simulink subsystem "Main"  (R2025b)
settings: Solver=VariableStepAuto  StartTime=0.0  StopTime=10.0  RelTol=1e-3
undefined symbols (not defined in the file): Aero_balance, Aeromaps_ON, air_density, Balance_R_11, Br_coef_of_friction_F, Br_coef_of_friction_R, Br_pistons_area_F, Br_pistons_area_R, CdA, CdA_R_11, ClA, ClA_R_11, CoG_z, Default_Fz_FL, Default_Fz_FR, Default_Fz_RL, Default_Fz_RR, Effective_br_disk_r_F, Effective_br_disk_r_R, Front_brake_balance, Front_brake_pump_area, Front_desired_brake_p_balance, Fx, Fy, Fz, g, Gear_ratio, Iz_wehicle, Iz_wheel, Lf, LLTD, Lock_brake_balance, Lr, Mass, Motor_maximum_power, PRT_efficiency, Rear_brake_pump_area, Roll_Angle_11, SA, SR, start_acc_x, start_acc_y, start_velocity_x, start_velocity_y, start_yaw_acc, start_yaw_rate, Static_Camber_FL, Static_Camber_FR, Static_Camber_RL, Static_Camber_RR, Static_Toe_FL, Static_Toe_FR, Static_Toe_RL, Static_Toe_RR, Steering_Angle_FL, Steering_Angle_FR, Steering_Wheel_Angle, Tire_pressure_FL, Tire_pressure_FR, Tire_pressure_RL ... (+18)
libraries: simulink_extras x9, simulink x7
(part 2 of 3)

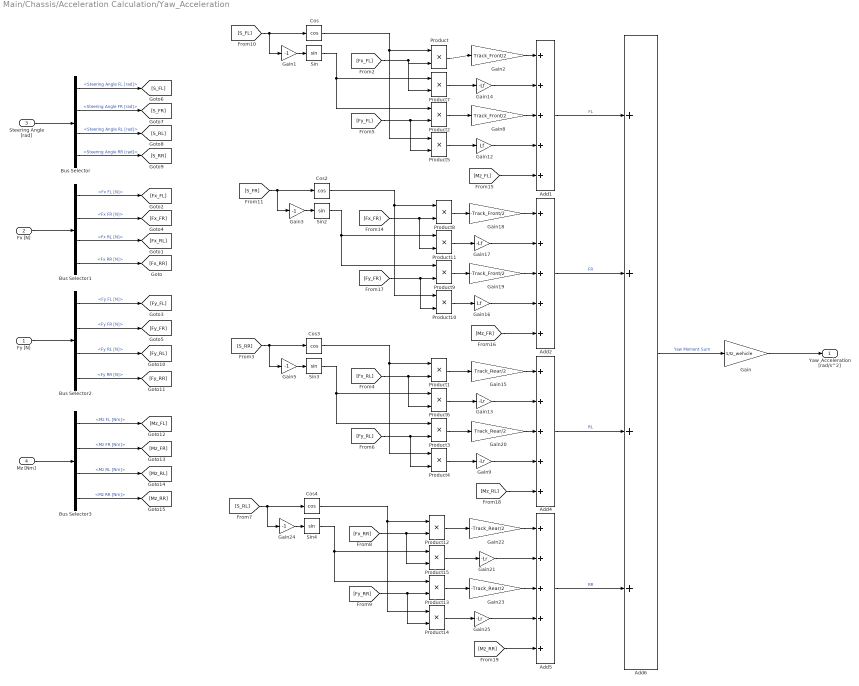
== system Main/Chassis/Acceleration Calculation/Yaw_Acceleration ==
  Fy [N] : Inport
  Fx [N] : Inport  Port=2
  Steering Angle [rad] : Inport  Port=3
  Mz [Nm] : Inport  Port=4
  Add{1..2,4..5} (4 alike) : Sum  Inputs=5
  Add6 : Sum  Inputs=4
  Bus Selector : BusSelector  OutputSignals=Steering Angle FL [rad],Steering Angle FR [rad],Steering Angle RL [rad],Steering Angle RR [rad]
  Bus Selector1 : BusSelector  OutputSignals=Fx FL [N],Fx FR [N],Fx RL [N],Fx RR [N]
  Bus Selector2 : BusSelector  OutputSignals=Fy FL [N],Fy FR [N],Fy RL [N],Fy RR [N]
  Bus Selector3 : BusSelector  OutputSignals=Mz FL [Nm],Mz FR [Nm],Mz RL [Nm],Mz RR [Nm]
  Cos{,2..4} (4 alike) : Trigonometry  Operator=cos
  Gain : Gain  Gain=1/Iz_wehicle
  Gain{1,3,5,24} (4 alike) : Gain  Gain=-1
  Gain12 : Gain  Gain=Lf
  Gain{9,13,21,25} (4 alike) : Gain  Gain=-Lr
  Gain14 : Gain  Gain=-Lf
  Gain15 : Gain  Gain=Track_Rear/2
  Gain16 : Gain  Gain=Lf
  Gain17 : Gain  Gain=-Lf
  Gain18 : Gain  Gain=-Track_Front/2
  Gain19 : Gain  Gain=-Track_Front/2
  Gain2 : Gain  Gain=Track_Front/2
  Gain20 : Gain  Gain=Track_Rear/2
  Gain22 : Gain  Gain=-Track_Rear/2
  Gain23 : Gain  Gain=-Track_Rear/2
  Gain8 : Gain  Gain=Track_Front/2
  Product{,1..15} (16 alike) : Product
  Sin{,2..4} (4 alike) : Trigonometry
  Yaw_Acceleration [rad/s^2] : Outport
  wires:
  Add1/1 -> Add6/1  "FL"
  Add5/1 -> Add6/4  "RR"
  Add2/1 -> Add6/2  "FR"
  Add4/1 -> Add6/3  "RL"
  [Mz_RR] -> Add5/5
  [Mz_RL] -> Add4/5
  [Mz_FR] -> Add2/5
  [Mz_FL] -> Add1/5
  Bus Selector3/2 -> [Mz_FR]  "<Mz FR [Nm]>"
  Bus Selector3/4 -> [Mz_RR]  "<Mz RR [Nm]>"
  Bus Selector3/3 -> [Mz_RL]  "<Mz RL [Nm]>"
  Bus Selector3/1 -> [Mz_FL]  "<Mz FL [Nm]>"
  Cos4/1 -> Product12/1, Product14/1
  Gain23/1 -> Add5/3
  [Fx_RR] -> Product12/2, Product15/2
  Gain22/1 -> Add5/1
  Gain21/1 -> Add5/2
  [Fy_RR] -> Product14/2, Product13/2
  [S_RL] -> Gain24/1, Cos4/1
  Gain25/1 -> Add5/4
  Gain24/1 -> Sin4/1
  Product13/1 -> Gain23/1
  Product12/1 -> Gain22/1
  Product14/1 -> Gain25/1
  Sin4/1 -> Product13/1, Product15/1
  Product15/1 -> Gain21/1
  Cos3/1 -> Product1/1, Product4/1
  Sin3/1 -> Product3/1, Product6/1
  Product4/1 -> Gain9/1
  Gain5/1 -> Sin3/1
  Product3/1 -> Gain20/1
  Product1/1 -> Gain15/1
  Product6/1 -> Gain13/1
  Gain9/1 -> Add4/4
  Gain20/1 -> Add4/3
  Gain13/1 -> Add4/2
  Gain15/1 -> Add4/1
  [Fx_RL] -> Product6/2, Product1/2
  [Fy_RL] -> Product4/2, Product3/2
  [S_RR] -> Cos3/1, Gain5/1
  Cos2/1 -> Product8/1, Product10/1
  Sin2/1 -> Product9/1, Product11/1
  Product10/1 -> Gain16/1
  Gain3/1 -> Sin2/1
  Product9/1 -> Gain19/1
  Product8/1 -> Gain18/1
  Product11/1 -> Gain17/1
  Gain16/1 -> Add2/4
  Gain19/1 -> Add2/3
  Gain17/1 -> Add2/2
  Gain18/1 -> Add2/1
  [Fx_FR] -> Product8/2, Product11/2
  [Fy_FR] -> Product10/2, Product9/2
  [S_FR] -> Cos2/1, Gain3/1
  Gain12/1 -> Add1/4
  Gain14/1 -> Add1/2
  Gain8/1 -> Add1/3
  Gain2/1 -> Add1/1
  Bus Selector/2 -> [S_FR]  "<Steering Angle FR [rad]>"
  [S_FL] -> Cos/1, Gain1/1
  Bus Selector/1 -> [S_FL]  "<Steering Angle FL [rad]>"
  Bus Selector/4 -> [S_RR]  "<Steering Angle RR [rad]>"
  Bus Selector/3 -> [S_RL]  "<Steering Angle RL [rad]>"
  Bus Selector2/2 -> [Fy_FR]  "<Fy FR [N]>"
  Bus Selector1/2 -> [Fx_FR]  "<Fx FR [N]>"
  [Fy_FL] -> Product5/2, Product2/2
  Bus Selector2/1 -> [Fy_FL]  "<Fy FL [N]>"
  [Fx_FL] -> Product7/2, Product/2
  Bus Selector1/1 -> [Fx_FL]  "<Fx FL [N]>"
  Mz [Nm]/1 -> Bus Selector3/1
  Product5/1 -> Gain12/1
  Sin/1 -> Product2/1, Product7/1
  Product/1 -> Gain2/1
  Product2/1 -> Gain8/1
  Bus Selector2/4 -> [Fy_RR]  "<Fy RR [N]>"
  Fx [N]/1 -> Bus Selector1/1
  Product7/1 -> Gain14/1
  Cos/1 -> Product/1, Product5/1
  Bus Selector1/3 -> [Fx_RL]  "<Fx RL [N]>"
  Fy [N]/1 -> Bus Selector2/1
  Bus Selector2/3 -> [Fy_RL]  "<Fy RL [N]>"
  Gain1/1 -> Sin/1
  Steering Angle [rad]/1 -> Bus Selector/1
  Bus Selector1/4 -> [Fx_RR]  "<Fx RR [N]>"
  Add6/1 -> Gain/1  "Yaw Moment Sum"
  Gain/1 -> Yaw_Acceleration [rad/s^2]/1

== system Main/Powertrain/Motors/Control Algorithms ==
  Motor Torque after FW [Nm] : Inport
  Torque Command [Nm] : Inport  Port=2
  Wheel Speed [rad/s] : Inport  Port=3
  Bus Creator : BusCreator  Inputs=4
  Bus Selector : BusSelector  OutputSignals=Motor Torque FL after FW [Nm],Motor Torque FR after FW [Nm],Motor Torque RL after FW [Nm],Motor Torque RR after FW [Nm]
  Constant : Constant  Value=TV_ON
  Gain : Gain
  Gain1 : Gain
  Switch{,1..3} (4 alike) : Switch  Criteria=u2 > Threshold  SaturateOnIntegerOverflow=off  InputSameDT=off
  TV Algorithm : Subsystem
  Motor Torque after TV [Nm] : Outport
  wires:
  Wheel Speed [rad/s]/1 -> TV Algorithm/2(Wheel Speed [rad/s])
  Gain1/1 -> Switch3/3
  Gain/1 -> Switch2/3
  Torque Command [Nm]/1 -> TV Algorithm/1(Torque Command [Nm])
  TV Algorithm/4(Commanded Torque RR [Nm]) -> Switch3/1  "Motor Torque RR"
  TV Algorithm/3(Commanded Torque RL [Nm]) -> Switch2/1  "Motor Torque RL"
  TV Algorithm/2(Commanded Torque FR [Nm]) -> Switch1/1
  TV Algorithm/1(Commanded Torque FL [Nm]) -> Switch/1
  Switch1/1 -> Bus Creator/2  "Motor Torque FR after TV [Nm]"
  Switch/1 -> Bus Creator/1  "Motor Torque FL after TV [Nm]"
  Bus Creator/1 -> Motor Torque after TV [Nm]/1  "Motor Torque after TV [Nm]"
  Switch2/1 -> Bus Creator/3  "Motor Torque RL after TV [Nm]"
  Switch3/1 -> Bus Creator/4  "Motor Torque RR after TV [Nm]"
  Bus Selector/4 -> Gain1/1  "<Motor Torque RR after FW [Nm]>"
  Bus Selector/3 -> Gain/1  "<Motor Torque RL after FW [Nm]>"
  Bus Selector/2 -> Switch1/3  "<Motor Torque FR after FW [Nm]>"
  Bus Selector/1 -> Switch/3  "<Motor Torque FL after FW [Nm]>"
  Motor Torque after FW [Nm]/1 -> Bus Selector/1
  Constant/1 -> Switch/2, Switch1/2, Switch2/2, Switch3/2

== system Main/Powertrain/Motors/Field Weakening ==
  Torque Command [Nm] : Inport
  Wheel Speed [rad/s] : Inport  Port=2
  Bus Creator : BusCreator  Inputs=4
  Bus Selector : BusSelector  OutputSignals=Wheel Speed FL [rad/s],Wheel Speed FR [rad/s],Wheel Speed RL [rad/s],Wheel Speed RR [rad/s]
  Constant : Constant  Value=Motor_maximum_power
  Gain : Gain  Gain=0
  Gain{1..2,5,7} (4 alike) : Gain  Gain=-1
  Gain10 : Gain
  Gain11 : Gain
  Gain{3..4,6,8} (4 alike) : Gain  Gain=Gear_ratio
  Gain9 : Gain  Gain=0
  Product : Product  Inputs=*/
  Product1 : Product  Inputs=/*
  Product2 : Product  Inputs=/*
  Product3 : Product  Inputs=*/
  Saturation Dynamic{,1..3} (4 alike) : simulink/Discontinuities/Saturation Dynamic  OutMin=[]  OutMax=[]  OutDataTypeStr=Inherit: Same as second input  OutDataType=fixdt(1, 16)  OutScaling=2^-10  DoSatur=off
  Motor Torque after FW [Nm] : Outport
  wires:
  Gain2/1 -> Saturation Dynamic1/3
  Gain1/1 -> Saturation Dynamic/3
  Wheel Speed [rad/s]/1 -> Bus Selector/1
  Gain11/1 -> Bus Creator/2  "Motor Torque RL after FW [Nm]"
  Gain10/1 -> Bus Creator/3  "Motor Torque RR after FW [Nm]"
  Gain9/1 -> Bus Creator/4  "Motor Torque FR after FW [Nm]"
  Gain/1 -> Bus Creator/1  "Motor Torque FL after FW [Nm]"
  Bus Creator/1 -> Motor Torque after FW [Nm]/1  "Motor Torque after FW [Nm]"
  Saturation Dynamic3/1 -> Gain9/1
  Gain7/1 -> Saturation Dynamic3/3
  Product3/1 -> Saturation Dynamic3/1, Gain7/1  "Maximum Torque FR after FW [Nm]"
  Bus Selector/4 -> Gain8/1  "<Wheel Speed RR [rad/s]>"
  Gain8/1 -> Product3/2  "Motor Speed FR [rad/s]"
  Constant/1 -> Product3/1, Product/1, Product2/2, Product1/2
  Torque Command [Nm]/1 -> Saturation Dynamic1/2, Saturation Dynamic3/2, Saturation Dynamic/2, Saturation Dynamic2/2
  Gain5/1 -> Saturation Dynamic2/3
  Bus Selector/1 -> Gain6/1  "<Wheel Speed FL [rad/s]>"
  Product2/1 -> Saturation Dynamic2/1, Gain5/1  "Maximum Torque FL after FW [Nm]"
  Gain6/1 -> Product2/1  "Motor Speed FL [rad/s]"
  Saturation Dynamic2/1 -> Gain/1
  Saturation Dynamic/1 -> Gain11/1
  Gain4/1 -> Product/2  "Motor Speed RR [rad/s]"
  Gain3/1 -> Product1/1  "Motor Speed RL [rad/s]"
  Bus Selector/3 -> Gain4/1  "<Wheel Speed RL [rad/s]>"
  Product1/1 -> Gain1/1, Saturation Dynamic/1  "Maximum Torque RL after FW [Nm]"
  Bus Selector/2 -> Gain3/1  "<Wheel Speed FR [rad/s]>"
  Product/1 -> Gain2/1, Saturation Dynamic1/1  "Maximum Torque RR after FW [Nm]"
  Saturation Dynamic1/1 -> Gain10/1

== system Main/Powertrain/Motors/Power Limit ==
  Motor Torque after TV [Nm] : Inport
  "Torque Command {Nm]" : Inport  Port=2
  Wheel Speed [rad/s] : Inport  Port=3
  Bus Creator : BusCreator  Inputs=5
  Bus Selector : BusSelector  OutputSignals=Motor Torque FL after TV [Nm],Motor Torque FR after TV [Nm],Motor Torque RL after TV [Nm],Motor Torque RR after TV [Nm]
  Constant : Constant  Value=TV_ON
  Power Calculation : Subsystem
  Switch{,1..3} (4 alike) : Switch  Criteria=u2 > Threshold  SaturateOnIntegerOverflow=off  InputSameDT=off
  Motor Power [W] : Outport
  Motor Torque [Nm] : Outport  Port=2
  wires:
  Wheel Speed [rad/s]/1 -> Power Calculation/1(Wheel Speed [rad/s])
  "Torque Command {Nm]"/1 -> Bus Creator/5
  Bus Creator/1 -> Motor Torque [Nm]/1
  Constant/1 -> Switch1/2, Switch3/2, Switch2/2, Switch/2
  Bus Selector/1 -> Switch/3, Switch/1  "<Motor Torque FL after TV [Nm]>"
  Bus Selector/4 -> Switch3/3, Switch3/1  "<Motor Torque RR after TV [Nm]>"
  Bus Selector/3 -> Switch2/3, Switch2/1  "<Motor Torque RL after TV [Nm]>"
  Switch1/1 -> Bus Creator/2  "Motor Torque FR [Nm]"
  Switch/1 -> Bus Creator/1  "Motor Torque FL [Nm]"
  Switch2/1 -> Bus Creator/3  "Motor Torque RL [Nm]"
  Switch3/1 -> Bus Creator/4  "Motor Torque RR [Nm]"
  Bus Selector/2 -> Switch1/3, Switch1/1  "<Motor Torque FR after TV [Nm]>"
  Power Calculation/1(Motor Power [W]) -> Motor Power [W]/1
  Motor Torque after TV [Nm]/1 -> Power Calculation/2(Motor Torque after TV [Nm]), Bus Selector/1

== system Main/Powertrain/Motors/Regen Braking ==
  Brake Pressure Front [bar] : Inport
  Brake Pressure Rear [bar] : Inport  Port=2
  " " : Constant  Value=Front_desired_brake_p_balance
  AND : Logic  IconShape=distinctive  AllPortsSameDT=off  OutDataTypeStr=boolean
  Cast To Boolean : DataTypeConversion  OutDataTypeStr=double  SaturateOnIntegerOverflow=off  RndMeth=Floor
  Compare To Constant : simulink/Logic and Bit Operations/Compare To Constant  relop=>=  const=5  OutDataTypeStr=boolean
  Compare To Constant1 : simulink/Logic and Bit Operations/Compare To Constant  relop=>=  const=5  OutDataTypeStr=boolean
  Gain : Gain  Gain=-1
  Product1 : Product
  Saturation2 : Saturate  UpperLimit=29  LowerLimit=0
  Subsystem : Subsystem
  Torque_to_Current_Conversion : Lookup_n-D  NumberOfTableDimensions=1  BreakpointsForDimension1=[0 29]  Table=[0 44]  InternalRulePriority=Speed  RndMeth=Simplest
  Negative Torque Command [Nm] : Outport
  wires:
  Brake Pressure Front [bar]/1 -> Subsystem/1(Brake_Preasure_Front), Compare To Constant1/1
  Brake Pressure Rear [bar]/1 -> Subsystem/2(Brake_Preasure_Rear), Compare To Constant/1
  Gain/1 -> Negative Torque Command [Nm]/1  "Negative Torque Command [Nm]"
  Compare To Constant1/1 -> AND/1
  AND/1 -> Cast To Boolean/1
  Subsystem/1("Motor_Rear_\"Preasure\"") -> Torque_to_Current_Conversion/1
  Saturation2/1 -> Product1/2
  Product1/1 -> Gain/1
  Torque_to_Current_Conversion/1 -> Saturation2/1
  Cast To Boolean/1 -> Product1/1
  Compare To Constant/1 -> AND/2
  " "/1 -> Subsystem/3(Desired_Brake_Balance)  "Desired_Brake_Balance"

== system Main/Powertrain/Motors/Torque Command [Nm] ==
  APPS [%] : Inport
  Constant : Constant  Value=Torque_limit_set
  Merge : Merge  Inputs=11
  Switch Case : SwitchCase  CaseConditions={1,2,3,4,5,6,7,8,9,10}
  Switch Case Action Subsystem : Subsystem  TreatAsAtomicUnit=on
  Switch Case Action Subsystem1 : Subsystem  TreatAsAtomicUnit=on
  Switch Case Action Subsystem10 : Subsystem  TreatAsAtomicUnit=on
  Switch Case Action Subsystem2 : Subsystem  TreatAsAtomicUnit=on
  Switch Case Action Subsystem3 : Subsystem  TreatAsAtomicUnit=on
  Switch Case Action Subsystem4 : Subsystem  TreatAsAtomicUnit=on
  Switch Case Action Subsystem5 : Subsystem  TreatAsAtomicUnit=on
  Switch Case Action Subsystem6 : Subsystem  TreatAsAtomicUnit=on
  Switch Case Action Subsystem7 : Subsystem  TreatAsAtomicUnit=on
  Switch Case Action Subsystem8 : Subsystem  TreatAsAtomicUnit=on
  Switch Case Action Subsystem9 : Subsystem  TreatAsAtomicUnit=on
  Positive Torque Command [Nm] : Outport
  wires:
  Switch Case/8 -> Switch Case Action Subsystem3/Action
  Switch Case/3 -> Switch Case Action Subsystem8/Action
  Switch Case/4 -> Switch Case Action Subsystem7/Action
  Switch Case/5 -> Switch Case Action Subsystem6/Action
  Switch Case/10 -> Switch Case Action Subsystem1/Action
  Switch Case Action Subsystem/1(Out1) -> Merge/11
  Switch Case Action Subsystem2/1(Out1) -> Merge/9
  Switch Case Action Subsystem5/1(Out1) -> Merge/6
  Switch Case/6 -> Switch Case Action Subsystem5/Action
  Switch Case Action Subsystem3/1(Out1) -> Merge/8
  Switch Case Action Subsystem4/1(Out1) -> Merge/7
  Switch Case Action Subsystem6/1(Out1) -> Merge/5
  Switch Case Action Subsystem10/1(Out1) -> Merge/1
  Switch Case Action Subsystem9/1(Out1) -> Merge/2
  Switch Case/11 -> Switch Case Action Subsystem/Action
  Constant/1 -> Switch Case/1
  Switch Case/7 -> Switch Case Action Subsystem4/Action
  Switch Case Action Subsystem7/1(Out1) -> Merge/4
  Switch Case/9 -> Switch Case Action Subsystem2/Action
  Switch Case Action Subsystem1/1(Out1) -> Merge/10
  Merge/1 -> Positive Torque Command [Nm]/1
  Switch Case/1 -> Switch Case Action Subsystem10/Action
  Switch Case Action Subsystem8/1(Out1) -> Merge/3
  Switch Case/2 -> Switch Case Action Subsystem9/Action
  APPS [%]/1 -> Switch Case Action Subsystem/1(APPS), Switch Case Action Subsystem1/1(APPS), Switch Case Action Subsystem3/1(APPS), Switch Case Action Subsystem5/1(APPS), Switch Case Action Subsystem6/1(APPS), Switch Case Action Subsystem8/1(APPS), Switch Case Action Subsystem10/1(APPS), Switch Case Action Subsystem9/1(APPS), Switch Case Action Subsystem7/1(APPS), Switch Case Action Subsystem4/1(APPS), Switch Case Action Subsystem2/1(APPS)

== system Main/Wheels & Tires/Brakes/Brake_Balance_Adjustment ==
  Braking_Torque_F [Nm] : Inport
  Braking_Torque_R [Nm] : Inport  Port=2
  Add : Sum
  Add1 : Sum
  Add2 : Sum
  Compare To Constant1 : simulink/Logic and Bit Operations/Compare To Constant  relop=>  const=1  OutDataTypeStr=boolean
  Constant : Constant  Value=Lock_brake_balance
  Constant1 : Constant  Value=Lock_brake_balance
  Constant2 : Constant  Value=Front_brake_balance
  Enabled Subsystem : Subsystem  TreatAsAtomicUnit=on
  Product : Product  Inputs=*/
  Product1 : Product
  Subtract : Sum  Inputs=-+
  Subtract1 : Sum  Inputs=-+
  Switch : Switch  Threshold=1  SaturateOnIntegerOverflow=off  InputSameDT=off
  Switch1 : Switch  Threshold=1  SaturateOnIntegerOverflow=off  InputSameDT=off
  Terminator : Terminator
  Adj_Braking_Torque_F [Nm] : Outport
  Adj_Braking_Torque_R [Nm] : Outport  Port=2
  wires:
  Subtract/1 -> Switch1/3  "Locked_Torque_R"
  Add1/1 -> Switch/3  "Locked_Torque_F"
  Subtract1/1 -> Switch1/1  "Adjusted_Torque_R"
  Add2/1 -> Subtract1/2, Product1/2
  Braking_Torque_R [Nm]/1 -> Subtract/2, Add2/2
  Product1/1 -> Switch/1, Add1/2, Subtract/1, Subtract1/1  "Adjusted_Torque_F"
  Braking_Torque_F [Nm]/1 -> Add2/1, Add1/1
  Constant2/1 -> Product1/1
  Compare To Constant1/1 -> Enabled Subsystem/Enable
  Enabled Subsystem/1(Out1) -> Terminator/1  "Brake_balance"
  Product/1 -> Enabled Subsystem/1(In1)  "Brake_balance"
  Add/1 -> Product/2
  Constant1/1 -> Switch1/2
  Switch1/1 -> Adj_Braking_Torque_R [Nm]/1, Compare To Constant1/1, Add/2  "Adj_Rear"
  Switch/1 -> Add/1, Product/1, Adj_Braking_Torque_F [Nm]/1  "Adj_Front"
  Constant/1 -> Switch/2

== system Main/Wheels & Tires/Brakes/Braking_Torque_Front ==
  Brake_Pressure [bar] : Inport
  Gain : Gain  Gain=1e5
  Gain1 : Gain  Gain=Effective_br_disk_r_F
  Product : Product  Inputs=3
  coefficient of friction : Constant  Value=Br_coef_of_friction_F
  piston area : Constant  Value=Br_pistons_area_F
  Braking_torque [Nm] : Outport
  wires:
  Gain1/1 -> Braking_torque [Nm]/1  "Braking torque [Nm]"
  Product/1 -> Gain1/1  "Braking force [N]"
  piston area/1 -> Product/3
  coefficient of friction/1 -> Product/2
  Gain/1 -> Product/1  "[Pa]"
  Brake_Pressure [bar]/1 -> Gain/1  "[bar]"

== system Main/Wheels & Tires/Brakes/Braking_Torque_Rear ==
  Brake_Pressure [bar] : Inport
  Gain1 : Gain  Gain=1e5
  Gain2 : Gain  Gain=Effective_br_disk_r_R
  Product2 : Product  Inputs=3
  coefficient of friction : Constant  Value=Br_coef_of_friction_R
  piston area : Constant  Value=Br_pistons_area_R
  Braking_Torque [Nm] : Outport
  wires:
  Brake_Pressure [bar]/1 -> Gain1/1
  coefficient of friction/1 -> Product2/2
  Gain1/1 -> Product2/1  "[Pa]"
  Gain2/1 -> Braking_Torque [Nm]/1  "Braking_Torque [Nm]"
  piston area/1 -> Product2/3
  Product2/1 -> Gain2/1  "Braking_Force [N]"

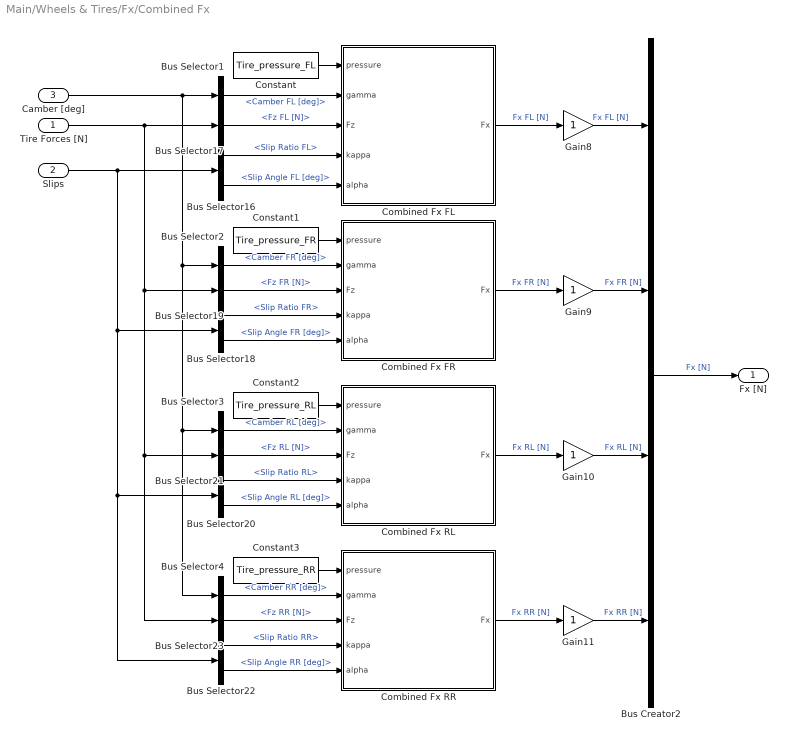
== system Main/Wheels & Tires/Fx/Combined Fx ==
  Tire Forces [N] : Inport
  Slips : Inport  Port=2
  Camber [deg] : Inport  Port=3
  Bus Creator2 : BusCreator  Inputs=4
  Bus Selector1 : BusSelector  OutputSignals=Camber FL [deg]
  Bus Selector16 : BusSelector  OutputSignals=Slip Ratio.Slip Ratio FL,Slip Angle [deg].Slip Angle FL [deg]
  Bus Selector17 : BusSelector  OutputSignals=Fz FL [N]
  Bus Selector18 : BusSelector  OutputSignals=Slip Ratio.Slip Ratio FR,Slip Angle [deg].Slip Angle FR [deg]
  Bus Selector19 : BusSelector  OutputSignals=Fz FR [N]
  Bus Selector2 : BusSelector  OutputSignals=Camber FR [deg]
  Bus Selector20 : BusSelector  OutputSignals=Slip Ratio.Slip Ratio RL,Slip Angle [deg].Slip Angle RL [deg]
  Bus Selector21 : BusSelector  OutputSignals=Fz RL [N]
  Bus Selector22 : BusSelector  OutputSignals=Slip Ratio.Slip Ratio RR,Slip Angle [deg].Slip Angle RR [deg]
  Bus Selector23 : BusSelector  OutputSignals=Fz RR [N]
  Bus Selector3 : BusSelector  OutputSignals=Camber RL [deg]
  Bus Selector4 : BusSelector  OutputSignals=Camber RR [deg]
  Combined Fx FL : MATLAB Function  TreatAsAtomicUnit=on
  Combined Fx FR : MATLAB Function  TreatAsAtomicUnit=on
  Combined Fx RL : MATLAB Function  TreatAsAtomicUnit=on
  Combined Fx RR : MATLAB Function  TreatAsAtomicUnit=on
  Constant : Constant  Value=Tire_pressure_FL
  Constant1 : Constant  Value=Tire_pressure_FR
  Constant2 : Constant  Value=Tire_pressure_RL
  Constant3 : Constant  Value=Tire_pressure_RR
  Gain{8..11} (4 alike) : Gain
  Fx [N] : Outport
  wires:
  Bus Selector4/1 -> Combined Fx RR/2(gamma)  "<Camber RR [deg]>"
  Bus Selector3/1 -> Combined Fx RL/2(gamma)  "<Camber RL [deg]>"
  Bus Selector2/1 -> Combined Fx FR/2(gamma)  "<Camber FR [deg]>"
  Bus Selector1/1 -> Combined Fx FL/2(gamma)  "<Camber FL [deg]>"
  Constant3/1 -> Combined Fx RR/1(pressure)
  Constant2/1 -> Combined Fx RL/1(pressure)
  Constant1/1 -> Combined Fx FR/1(pressure)
  Constant/1 -> Combined Fx FL/1(pressure)
  Camber [deg]/1 -> Bus Selector1/1, Bus Selector2/1, Bus Selector3/1, Bus Selector4/1
  Bus Creator2/1 -> Fx [N]/1  "Fx [N]"
  Bus Selector22/2 -> Combined Fx RR/5(alpha)  "<Slip Angle RR [deg]>"
  Bus Selector23/1 -> Combined Fx RR/3(Fz)  "<Fz RR [N]>"
  Bus Selector16/2 -> Combined Fx FL/5(alpha)  "<Slip Angle FL [deg]>"
  Bus Selector18/2 -> Combined Fx FR/5(alpha)  "<Slip Angle FR [deg]>"
  Bus Selector21/1 -> Combined Fx RL/3(Fz)  "<Fz RL [N]>"
  Combined Fx RL/1(Fx) -> Gain10/1  "Fx RL [N]"
  Combined Fx FL/1(Fx) -> Gain8/1  "Fx FL [N]"
  Combined Fx FR/1(Fx) -> Gain9/1  "Fx FR [N]"
  Combined Fx RR/1(Fx) -> Gain11/1  "Fx RR [N]"
  Bus Selector19/1 -> Combined Fx FR/3(Fz)  "<Fz FR [N]>"
  Gain10/1 -> Bus Creator2/3  "Fx RL [N]"
  Bus Selector16/1 -> Combined Fx FL/4(kappa)  "<Slip Ratio FL>"
  Gain8/1 -> Bus Creator2/1  "Fx FL [N]"
  Tire Forces [N]/1 -> Bus Selector23/1, Bus Selector21/1, Bus Selector19/1, Bus Selector17/1
  Bus Selector17/1 -> Combined Fx FL/3(Fz)  "<Fz FL [N]>"
  Bus Selector22/1 -> Combined Fx RR/4(kappa)  "<Slip Ratio RR>"
  Bus Selector18/1 -> Combined Fx FR/4(kappa)  "<Slip Ratio FR>"
  Bus Selector20/1 -> Combined Fx RL/4(kappa)  "<Slip Ratio RL>"
  Bus Selector20/2 -> Combined Fx RL/5(alpha)  "<Slip Angle RL [deg]>"
  Slips/1 -> Bus Selector22/1, Bus Selector20/1, Bus Selector18/1, Bus Selector16/1
  Gain9/1 -> Bus Creator2/2  "Fx FR [N]"
  Gain11/1 -> Bus Creator2/4  "Fx RR [N]"

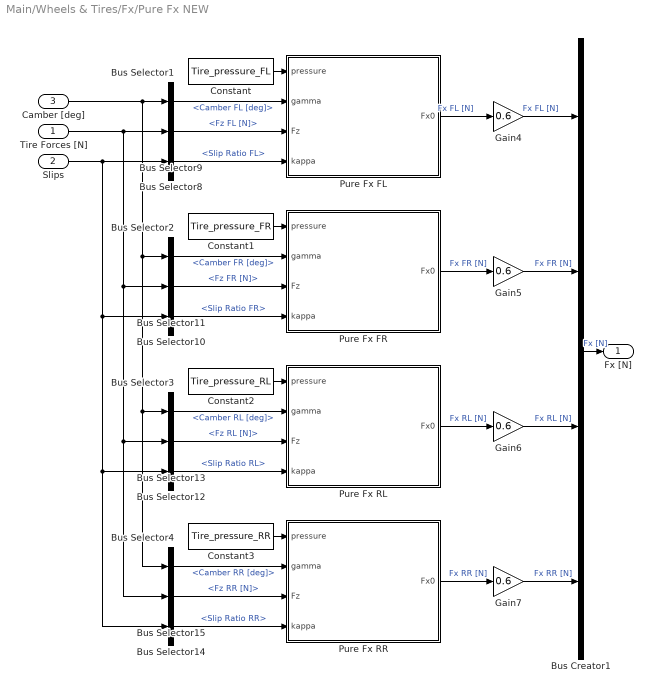
== system Main/Wheels & Tires/Fx/Pure Fx NEW ==
  Tire Forces [N] : Inport
  Slips : Inport  Port=2
  Camber [deg] : Inport  Port=3
  Bus Creator1 : BusCreator  Inputs=4
  Bus Selector1 : BusSelector  OutputSignals=Camber FL [deg]
  Bus Selector10 : BusSelector  OutputSignals=Slip Ratio.Slip Ratio FR
  Bus Selector11 : BusSelector  OutputSignals=Fz FR [N]
  Bus Selector12 : BusSelector  OutputSignals=Slip Ratio.Slip Ratio RL
  Bus Selector13 : BusSelector  OutputSignals=Fz RL [N]
  Bus Selector14 : BusSelector  OutputSignals=Slip Ratio.Slip Ratio RR
  Bus Selector15 : BusSelector  OutputSignals=Fz RR [N]
  Bus Selector2 : BusSelector  OutputSignals=Camber FR [deg]
  Bus Selector3 : BusSelector  OutputSignals=Camber RL [deg]
  Bus Selector4 : BusSelector  OutputSignals=Camber RR [deg]
  Bus Selector8 : BusSelector  OutputSignals=Slip Ratio.Slip Ratio FL
  Bus Selector9 : BusSelector  OutputSignals=Fz FL [N]
  Constant : Constant  Value=Tire_pressure_FL
  Constant1 : Constant  Value=Tire_pressure_FR
  Constant2 : Constant  Value=Tire_pressure_RL
  Constant3 : Constant  Value=Tire_pressure_RR
  Gain{4..7} (4 alike) : Gain  Gain=0.6
  Pure Fx FL : MATLAB Function  TreatAsAtomicUnit=on
  Pure Fx FR : MATLAB Function  TreatAsAtomicUnit=on
  Pure Fx RL : MATLAB Function  TreatAsAtomicUnit=on
  Pure Fx RR : MATLAB Function  TreatAsAtomicUnit=on
  Fx [N] : Outport
  wires:
  Bus Selector4/1 -> Pure Fx RR/2(gamma)  "<Camber RR [deg]>"
  Bus Selector3/1 -> Pure Fx RL/2(gamma)  "<Camber RL [deg]>"
  Bus Selector2/1 -> Pure Fx FR/2(gamma)  "<Camber FR [deg]>"
  Camber [deg]/1 -> Bus Selector1/1, Bus Selector2/1, Bus Selector3/1, Bus Selector4/1
  Bus Selector1/1 -> Pure Fx FL/2(gamma)  "<Camber FL [deg]>"
  Constant3/1 -> Pure Fx RR/1(pressure)
  Constant2/1 -> Pure Fx RL/1(pressure)
  Constant1/1 -> Pure Fx FR/1(pressure)
  Constant/1 -> Pure Fx FL/1(pressure)
  Gain6/1 -> Bus Creator1/3  "Fx RL [N]"
  Pure Fx RL/1(Fx0) -> Gain6/1  "Fx RL [N]"
  Gain7/1 -> Bus Creator1/4  "Fx RR [N]"
  Pure Fx FL/1(Fx0) -> Gain4/1  "Fx FL [N]"
  Bus Selector9/1 -> Pure Fx FL/3(Fz)  "<Fz FL [N]>"
  Bus Selector12/1 -> Pure Fx RL/4(kappa)  "<Slip Ratio RL>"
  Bus Creator1/1 -> Fx [N]/1  "Fx [N]"
  Bus Selector13/1 -> Pure Fx RL/3(Fz)  "<Fz RL [N]>"
  Gain5/1 -> Bus Creator1/2  "Fx FR [N]"
  Bus Selector10/1 -> Pure Fx FR/4(kappa)  "<Slip Ratio FR>"
  Gain4/1 -> Bus Creator1/1  "Fx FL [N]"
  Bus Selector11/1 -> Pure Fx FR/3(Fz)  "<Fz FR [N]>"
  Bus Selector14/1 -> Pure Fx RR/4(kappa)  "<Slip Ratio RR>"
  Bus Selector15/1 -> Pure Fx RR/3(Fz)  "<Fz RR [N]>"
  Tire Forces [N]/1 -> Bus Selector9/1, Bus Selector11/1, Bus Selector13/1, Bus Selector15/1
  Pure Fx RR/1(Fx0) -> Gain7/1  "Fx RR [N]"
  Pure Fx FR/1(Fx0) -> Gain5/1  "Fx FR [N]"
  Slips/1 -> Bus Selector8/1, Bus Selector12/1, Bus Selector14/1, Bus Selector10/1
  Bus Selector8/1 -> Pure Fx FL/4(kappa)  "<Slip Ratio FL>"

== system Main/Wheels & Tires/Fx/Pure Fx OLD ==
  Tire Forces [N] : Inport
  Slips : Inport  Port=2
  2-D Lookup Table1 : Lookup_n-D  BreakpointsForDimension1=Fz  BreakpointsForDimension2=SR  Table=Fx  UseLastTableValue=on  ApplyAccurateEfficientRounding=on  InternalRulePriority=Speed  RndMeth=Simplest
      settings: InputPortMap=u0,u1
  2-D Lookup Table2 : Lookup_n-D  BreakpointsForDimension1=Fz  BreakpointsForDimension2=SR  Table=Fx  UseLastTableValue=on  ApplyAccurateEfficientRounding=on  InternalRulePriority=Speed  RndMeth=Simplest
      settings: InputPortMap=u0,u1
  2-D Lookup Table3 : Lookup_n-D  BreakpointsForDimension1=Fz  BreakpointsForDimension2=SR  Table=Fx  ExtrapMethod=Clip  UseLastTableValue=on  ApplyAccurateEfficientRounding=on  InternalRulePriority=Speed  RndMeth=Simplest
      settings: InputPortMap=u0,u1
  2-D Lookup Table4 : Lookup_n-D  BreakpointsForDimension1=Fz  BreakpointsForDimension2=SR  Table=Fx  ExtrapMethod=Clip  UseLastTableValue=on  ApplyAccurateEfficientRounding=on  InternalRulePriority=Speed  RndMeth=Simplest
      settings: InputPortMap=u0,u1
  Bus Creator : BusCreator  Inputs=4
  Bus Selector : BusSelector  OutputSignals=Slip Ratio.Slip Ratio FL
  Bus Selector1 : BusSelector  OutputSignals=Fz FL [N]
  Bus Selector2 : BusSelector  OutputSignals=Slip Ratio.Slip Ratio FR
  Bus Selector3 : BusSelector  OutputSignals=Fz FR [N]
  Bus Selector4 : BusSelector  OutputSignals=Slip Ratio.Slip Ratio RL
  Bus Selector5 : BusSelector  OutputSignals=Fz RL [N]
  Bus Selector6 : BusSelector  OutputSignals=Slip Ratio.Slip Ratio RR
  Bus Selector7 : BusSelector  OutputSignals=Fz RR [N]
  Gain : Gain  Gain=0.8
  Gain1 : Gain  Gain=0.8
  Gain2 : Gain  Gain=1.6
  Gain3 : Gain  Gain=1.6
  Fx [N] : Outport
  wires:
  Bus Creator/1 -> Fx [N]/1  "Fx [N]"
  Gain2/1 -> Bus Creator/3  "Fx RL [N]"
  Bus Selector7/1 -> 2-D Lookup Table4/1  "<Fz RR [N]>"
  Bus Selector6/1 -> 2-D Lookup Table4/2  "<Slip Ratio RR>"
  Bus Selector4/1 -> 2-D Lookup Table3/2  "<Slip Ratio RL>"
  Bus Selector3/1 -> 2-D Lookup Table2/1  "<Fz FR [N]>"
  Slips/1 -> Bus Selector/1, Bus Selector2/1, Bus Selector4/1, Bus Selector6/1
  2-D Lookup Table1/1 -> Gain/1  "Fx FL [N]"
  Bus Selector1/1 -> 2-D Lookup Table1/1  "<Fz FL [N]>"
  Bus Selector/1 -> 2-D Lookup Table1/2  "<Slip Ratio FL>"
  2-D Lookup Table4/1 -> Gain3/1  "Fx RR [N]"
  Bus Selector5/1 -> 2-D Lookup Table3/1  "<Fz RL [N]>"
  Gain/1 -> Bus Creator/1  "Fx FL [N]"
  Gain1/1 -> Bus Creator/2  "Fx FR [N]"
  Bus Selector2/1 -> 2-D Lookup Table2/2  "<Slip Ratio FR>"
  Tire Forces [N]/1 -> Bus Selector3/1, Bus Selector5/1, Bus Selector7/1, Bus Selector1/1
  Gain3/1 -> Bus Creator/4  "Fx RR [N]"
  2-D Lookup Table3/1 -> Gain2/1  "Fx RL [N]"
  2-D Lookup Table2/1 -> Gain1/1  "Fx FR [N]"

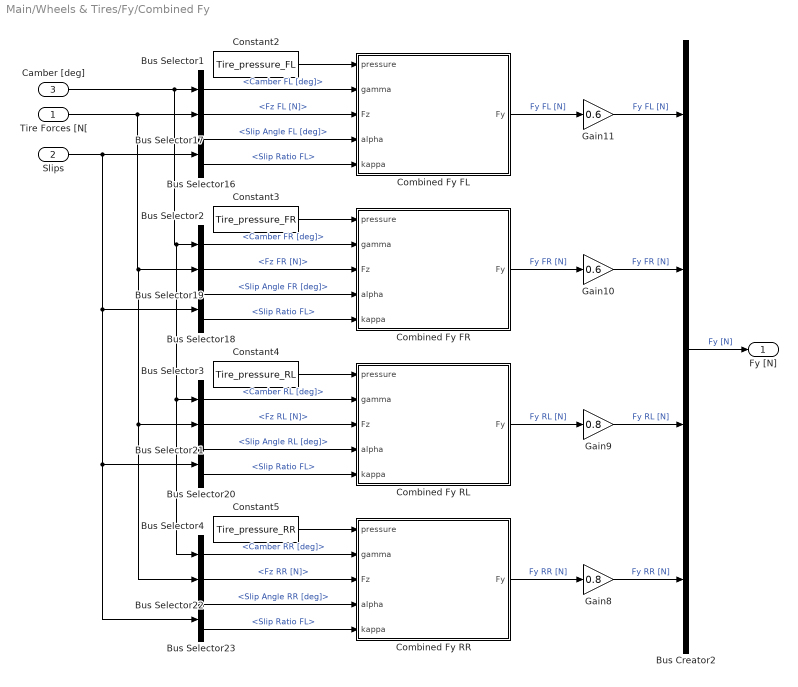
== system Main/Wheels & Tires/Fy/Combined Fy ==
  Tire Forces [N[ : Inport
  Slips : Inport  Port=2
  Camber [deg] : Inport  Port=3
  Bus Creator2 : BusCreator  Inputs=4
  Bus Selector1 : BusSelector  OutputSignals=Camber FL [deg]
  Bus Selector16 : BusSelector  OutputSignals=Slip Angle [deg].Slip Angle FL [deg],Slip Ratio.Slip Ratio FL
  Bus Selector17 : BusSelector  OutputSignals=Fz FL [N]
  Bus Selector18 : BusSelector  OutputSignals=Slip Angle [deg].Slip Angle FR [deg],Slip Ratio.Slip Ratio FL
  Bus Selector19 : BusSelector  OutputSignals=Fz FR [N]
  Bus Selector2 : BusSelector  OutputSignals=Camber FR [deg]
  Bus Selector20 : BusSelector  OutputSignals=Slip Angle [deg].Slip Angle RL [deg],Slip Ratio.Slip Ratio FL
  Bus Selector21 : BusSelector  OutputSignals=Fz RL [N]
  Bus Selector22 : BusSelector  OutputSignals=Fz RR [N]
  Bus Selector23 : BusSelector  OutputSignals=Slip Angle [deg].Slip Angle RR [deg],Slip Ratio.Slip Ratio FL
  Bus Selector3 : BusSelector  OutputSignals=Camber RL [deg]
  Bus Selector4 : BusSelector  OutputSignals=Camber RR [deg]
  Combined Fy FL : MATLAB Function  TreatAsAtomicUnit=on
  Combined Fy FR : MATLAB Function  TreatAsAtomicUnit=on
  Combined Fy RL : MATLAB Function  TreatAsAtomicUnit=on
  Combined Fy RR : MATLAB Function  TreatAsAtomicUnit=on  SystemSampleTime=0.001
  Constant2 : Constant  Value=Tire_pressure_FL
  Constant3 : Constant  Value=Tire_pressure_FR
  Constant4 : Constant  Value=Tire_pressure_RL
  Constant5 : Constant  Value=Tire_pressure_RR
  Gain10 : Gain  Gain=0.6
  Gain11 : Gain  Gain=0.6
  Gain8 : Gain  Gain=0.8
  Gain9 : Gain  Gain=0.8
  Fy [N] : Outport
  wires:
  Bus Selector4/1 -> Combined Fy RR/2(gamma)  "<Camber RR [deg]>"
  Bus Selector3/1 -> Combined Fy RL/2(gamma)  "<Camber RL [deg]>"
  Bus Selector2/1 -> Combined Fy FR/2(gamma)  "<Camber FR [deg]>"
  Camber [deg]/1 -> Bus Selector1/1, Bus Selector3/1, Bus Selector4/1, Bus Selector2/1
  Bus Selector1/1 -> Combined Fy FL/2(gamma)  "<Camber FL [deg]>"
  Bus Creator2/1 -> Fy [N]/1  "Fy [N]"
  Constant5/1 -> Combined Fy RR/1(pressure)
  Constant4/1 -> Combined Fy RL/1(pressure)
  Bus Selector22/1 -> Combined Fy RR/3(Fz)  "<Fz RR [N]>"
  Bus Selector19/1 -> Combined Fy FR/3(Fz)  "<Fz FR [N]>"
  Combined Fy FL/1(Fy) -> Gain11/1  "Fy FL [N]"
  Bus Selector23/1 -> Combined Fy RR/4(alpha)  "<Slip Angle RR [deg]>"
  Bus Selector17/1 -> Combined Fy FL/3(Fz)  "<Fz FL [N]>"
  Gain11/1 -> Bus Creator2/1  "Fy FL [N]"
  Bus Selector20/2 -> Combined Fy RL/5(kappa)  "<Slip Ratio FL>"
  Bus Selector21/1 -> Combined Fy RL/3(Fz)  "<Fz RL [N]>"
  Bus Selector18/2 -> Combined Fy FR/5(kappa)  "<Slip Ratio FL>"
  Combined Fy RL/1(Fy) -> Gain9/1  "Fy RL [N]"
  Bus Selector20/1 -> Combined Fy RL/4(alpha)  "<Slip Angle RL [deg]>"
  Gain10/1 -> Bus Creator2/2  "Fy FR [N]"
  Combined Fy RR/1(Fy) -> Gain8/1  "Fy RR [N]"
  Bus Selector23/2 -> Combined Fy RR/5(kappa)  "<Slip Ratio FL>"
  Constant3/1 -> Combined Fy FR/1(pressure)
  Bus Selector18/1 -> Combined Fy FR/4(alpha)  "<Slip Angle FR [deg]>"
  Bus Selector16/2 -> Combined Fy FL/5(kappa)  "<Slip Ratio FL>"
  Tire Forces [N[/1 -> Bus Selector19/1, Bus Selector21/1, Bus Selector22/1, Bus Selector17/1
  Combined Fy FR/1(Fy) -> Gain10/1  "Fy FR [N]"
  Slips/1 -> Bus Selector16/1, Bus Selector18/1, Bus Selector20/1, Bus Selector23/1
  Bus Selector16/1 -> Combined Fy FL/4(alpha)  "<Slip Angle FL [deg]>"
  Gain8/1 -> Bus Creator2/4  "Fy RR [N]"
  Gain9/1 -> Bus Creator2/3  "Fy RL [N]"
  Constant2/1 -> Combined Fy FL/1(pressure)

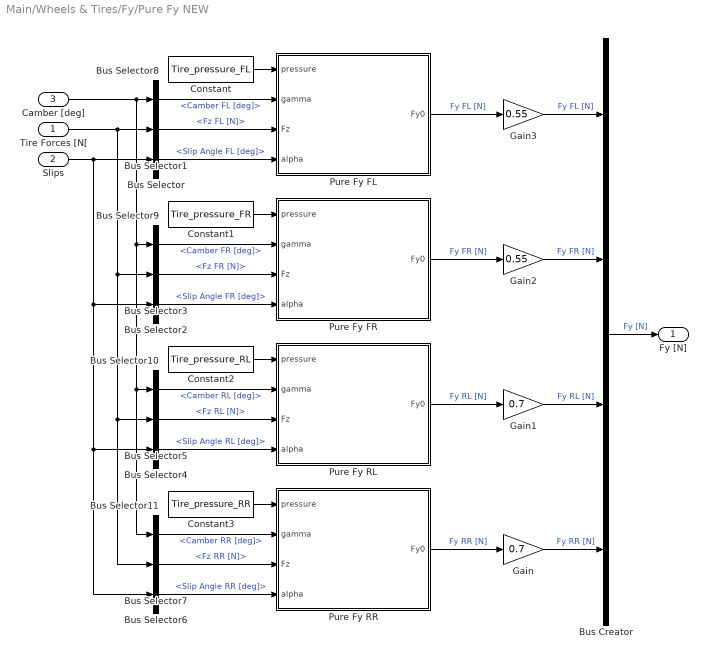
== system Main/Wheels & Tires/Fy/Pure Fy NEW ==
  Tire Forces [N[ : Inport
  Slips : Inport  Port=2
  Camber [deg] : Inport  Port=3
  Bus Creator : BusCreator  Inputs=4
  Bus Selector : BusSelector  OutputSignals=Slip Angle [deg].Slip Angle FL [deg]
  Bus Selector1 : BusSelector  OutputSignals=Fz FL [N]
  Bus Selector10 : BusSelector  OutputSignals=Camber RL [deg]
  Bus Selector11 : BusSelector  OutputSignals=Camber RR [deg]
  Bus Selector2 : BusSelector  OutputSignals=Slip Angle [deg].Slip Angle FR [deg]
  Bus Selector3 : BusSelector  OutputSignals=Fz FR [N]
  Bus Selector4 : BusSelector  OutputSignals=Slip Angle [deg].Slip Angle RL [deg]
  Bus Selector5 : BusSelector  OutputSignals=Fz RL [N]
  Bus Selector6 : BusSelector  OutputSignals=Slip Angle [deg].Slip Angle RR [deg]
  Bus Selector7 : BusSelector  OutputSignals=Fz RR [N]
  Bus Selector8 : BusSelector  OutputSignals=Camber FL [deg]
  Bus Selector9 : BusSelector  OutputSignals=Camber FR [deg]
  Constant : Constant  Value=Tire_pressure_FL
  Constant1 : Constant  Value=Tire_pressure_FR
  Constant2 : Constant  Value=Tire_pressure_RL
  Constant3 : Constant  Value=Tire_pressure_RR
  Gain : Gain  Gain=0.7
  Gain1 : Gain  Gain=0.7
  Gain2 : Gain  Gain=0.55
  Gain3 : Gain  Gain=0.55
  Pure Fy FL : MATLAB Function  TreatAsAtomicUnit=on
  Pure Fy FR : MATLAB Function  TreatAsAtomicUnit=on
  Pure Fy RL : MATLAB Function  TreatAsAtomicUnit=on
  Pure Fy RR : MATLAB Function  TreatAsAtomicUnit=on  SystemSampleTime=0.001
  Fy [N] : Outport
  wires:
  Bus Selector11/1 -> Pure Fy RR/2(gamma)  "<Camber RR [deg]>"
  Bus Selector10/1 -> Pure Fy RL/2(gamma)  "<Camber RL [deg]>"
  Bus Selector9/1 -> Pure Fy FR/2(gamma)  "<Camber FR [deg]>"
  Camber [deg]/1 -> Bus Selector8/1, Bus Selector9/1, Bus Selector10/1, Bus Selector11/1
  Bus Selector8/1 -> Pure Fy FL/2(gamma)  "<Camber FL [deg]>"
  Constant3/1 -> Pure Fy RR/1(pressure)
  Constant2/1 -> Pure Fy RL/1(pressure)
  Constant1/1 -> Pure Fy FR/1(pressure)
  Constant/1 -> Pure Fy FL/1(pressure)
  Bus Selector2/1 -> Pure Fy FR/4(alpha)  "<Slip Angle FR [deg]>"
  Bus Selector6/1 -> Pure Fy RR/4(alpha)  "<Slip Angle RR [deg]>"
  Gain3/1 -> Bus Creator/1  "Fy FL [N]"
  Bus Selector/1 -> Pure Fy FL/4(alpha)  "<Slip Angle FL [deg]>"
  Bus Selector7/1 -> Pure Fy RR/3(Fz)  "<Fz RR [N]>"
  Bus Selector4/1 -> Pure Fy RL/4(alpha)  "<Slip Angle RL [deg]>"
  Pure Fy FR/1(Fy0) -> Gain2/1  "Fy FR [N]"
  Bus Selector1/1 -> Pure Fy FL/3(Fz)  "<Fz FL [N]>"
  Gain2/1 -> Bus Creator/2  "Fy FR [N]"
  Slips/1 -> Bus Selector6/1, Bus Selector4/1, Bus Selector2/1, Bus Selector/1
  Pure Fy FL/1(Fy0) -> Gain3/1  "Fy FL [N]"
  Bus Selector3/1 -> Pure Fy FR/3(Fz)  "<Fz FR [N]>"
  Bus Creator/1 -> Fy [N]/1  "Fy [N]"
  Bus Selector5/1 -> Pure Fy RL/3(Fz)  "<Fz RL [N]>"
  Pure Fy RR/1(Fy0) -> Gain/1  "Fy RR [N]"
  Gain1/1 -> Bus Creator/3  "Fy RL [N]"
  Pure Fy RL/1(Fy0) -> Gain1/1  "Fy RL [N]"
  Gain/1 -> Bus Creator/4  "Fy RR [N]"
  Tire Forces [N[/1 -> Bus Selector3/1, Bus Selector5/1, Bus Selector7/1, Bus Selector1/1

== system Main/Wheels & Tires/Fy/Pure Fy OLD ==
  Tire Forces [N[ : Inport
  Slips : Inport  Port=2
  2-D Lookup Table{1..4} (4 alike) : Lookup_n-D  BreakpointsForDimension1=Fz  BreakpointsForDimension2=SA  Table=Fy  UseLastTableValue=on  ApplyAccurateEfficientRounding=on  InternalRulePriority=Speed  RndMeth=Simplest
      settings: InputPortMap=u0,u1
  Bus Creator1 : BusCreator  Inputs=4
  Bus Selector10 : BusSelector  OutputSignals=Slip Angle [deg].Slip Angle FR [deg]
  Bus Selector11 : BusSelector  OutputSignals=Fz FR [N]
  Bus Selector12 : BusSelector  OutputSignals=Slip Angle [deg].Slip Angle RL [deg]
  Bus Selector13 : BusSelector  OutputSignals=Fz RL [N]
  Bus Selector14 : BusSelector  OutputSignals=Slip Angle [deg].Slip Angle RR [deg]
  Bus Selector15 : BusSelector  OutputSignals=Fz RR [N]
  Bus Selector8 : BusSelector  OutputSignals=Slip Angle [deg].Slip Angle FL [deg]
  Bus Selector9 : BusSelector  OutputSignals=Fz FL [N]
  Gain{4..7} (4 alike) : Gain  Gain=0.8
  Fy [N] : Outport
  wires:
  Bus Creator1/1 -> Fy [N]/1  "Fy [N]"
  Gain5/1 -> Bus Creator1/3  "Fy RL [N]"
  2-D Lookup Table2/1 -> Gain6/1  "Fy FR [N]"
  2-D Lookup Table1/1 -> Gain7/1  "Fy FL [N]"
  Gain6/1 -> Bus Creator1/2  "Fy FR [N]"
  Bus Selector14/1 -> 2-D Lookup Table4/2  "<Slip Angle RR [deg]>"
  2-D Lookup Table4/1 -> Gain4/1  "Fy RR [N]"
  Bus Selector15/1 -> 2-D Lookup Table4/1  "<Fz RR [N]>"
  2-D Lookup Table3/1 -> Gain5/1  "Fy RL [N]"
  Bus Selector11/1 -> 2-D Lookup Table2/1  "<Fz FR [N]>"
  Bus Selector12/1 -> 2-D Lookup Table3/2  "<Slip Angle RL [deg]>"
  Bus Selector13/1 -> 2-D Lookup Table3/1  "<Fz RL [N]>"
  Tire Forces [N[/1 -> Bus Selector11/1, Bus Selector13/1, Bus Selector15/1, Bus Selector9/1
  Gain7/1 -> Bus Creator1/1  "Fy FL [N]"
  Bus Selector10/1 -> 2-D Lookup Table2/2  "<Slip Angle FR [deg]>"
  Bus Selector8/1 -> 2-D Lookup Table1/2  "<Slip Angle FL [deg]>"
  Gain4/1 -> Bus Creator1/4  "Fy RR [N]"
  Bus Selector9/1 -> 2-D Lookup Table1/1  "<Fz FL [N]>"
  Slips/1 -> Bus Selector10/1, Bus Selector12/1, Bus Selector14/1, Bus Selector8/1

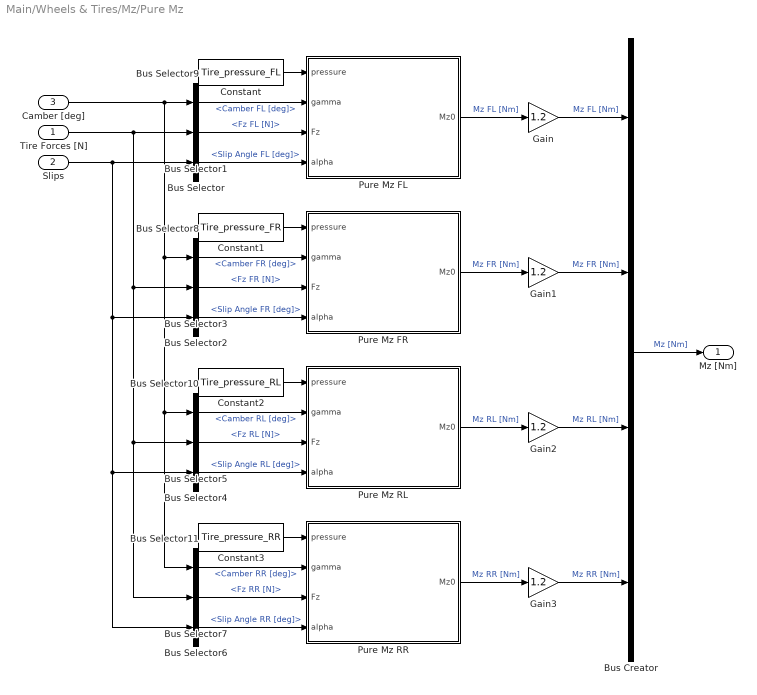
== system Main/Wheels & Tires/Mz/Pure Mz ==
  Tire Forces [N] : Inport
  Slips : Inport  Port=2
  Camber [deg] : Inport  Port=3
  Bus Creator : BusCreator  Inputs=4
  Bus Selector : BusSelector  OutputSignals=Slip Angle [deg].Slip Angle FL [deg]
  Bus Selector1 : BusSelector  OutputSignals=Fz FL [N]
  Bus Selector10 : BusSelector  OutputSignals=Camber RL [deg]
  Bus Selector11 : BusSelector  OutputSignals=Camber RR [deg]
  Bus Selector2 : BusSelector  OutputSignals=Slip Angle [deg].Slip Angle FR [deg]
  Bus Selector3 : BusSelector  OutputSignals=Fz FR [N]
  Bus Selector4 : BusSelector  OutputSignals=Slip Angle [deg].Slip Angle RL [deg]
  Bus Selector5 : BusSelector  OutputSignals=Fz RL [N]
  Bus Selector6 : BusSelector  OutputSignals=Slip Angle [deg].Slip Angle RR [deg]
  Bus Selector7 : BusSelector  OutputSignals=Fz RR [N]
  Bus Selector8 : BusSelector  OutputSignals=Camber FR [deg]
  Bus Selector9 : BusSelector  OutputSignals=Camber FL [deg]
  Constant : Constant  Value=Tire_pressure_FL
  Constant1 : Constant  Value=Tire_pressure_FR
  Constant2 : Constant  Value=Tire_pressure_RL
  Constant3 : Constant  Value=Tire_pressure_RR
  Gain{,1..3} (4 alike) : Gain  Gain=1.2
  Pure Mz FL : MATLAB Function  TreatAsAtomicUnit=on
  Pure Mz FR : MATLAB Function  TreatAsAtomicUnit=on
  Pure Mz RL : MATLAB Function  TreatAsAtomicUnit=on
  Pure Mz RR : MATLAB Function  TreatAsAtomicUnit=on
  Mz [Nm] : Outport
  wires:
  Bus Selector9/1 -> Pure Mz FL/2(gamma)  "<Camber FL [deg]>"
  Bus Selector11/1 -> Pure Mz RR/2(gamma)  "<Camber RR [deg]>"
  Bus Selector10/1 -> Pure Mz RL/2(gamma)  "<Camber RL [deg]>"
  Bus Selector8/1 -> Pure Mz FR/2(gamma)  "<Camber FR [deg]>"
  Constant1/1 -> Pure Mz FR/1(pressure)
  Constant3/1 -> Pure Mz RR/1(pressure)
  Pure Mz FL/1(Mz0) -> Gain/1  "Mz FL [Nm]"
  Pure Mz FR/1(Mz0) -> Gain1/1  "Mz FR [Nm]"
  Gain/1 -> Bus Creator/1  "Mz FL [Nm]"
  Constant/1 -> Pure Mz FL/1(pressure)
  Pure Mz RL/1(Mz0) -> Gain2/1  "Mz RL [Nm]"
  Bus Selector3/1 -> Pure Mz FR/3(Fz)  "<Fz FR [N]>"
  Bus Selector2/1 -> Pure Mz FR/4(alpha)  "<Slip Angle FR [deg]>"
  Bus Selector1/1 -> Pure Mz FL/3(Fz)  "<Fz FL [N]>"
  Gain2/1 -> Bus Creator/3  "Mz RL [Nm]"
  Gain1/1 -> Bus Creator/2  "Mz FR [Nm]"
  Camber [deg]/1 -> Bus Selector9/1, Bus Selector8/1, Bus Selector10/1, Bus Selector11/1
  Bus Selector5/1 -> Pure Mz RL/3(Fz)  "<Fz RL [N]>"
  Gain3/1 -> Bus Creator/4  "Mz RR [Nm]"
  Pure Mz RR/1(Mz0) -> Gain3/1  "Mz RR [Nm]"
  Bus Selector/1 -> Pure Mz FL/4(alpha)  "<Slip Angle FL [deg]>"
  Bus Selector7/1 -> Pure Mz RR/3(Fz)  "<Fz RR [N]>"
  Constant2/1 -> Pure Mz RL/1(pressure)
  Slips/1 -> Bus Selector/1, Bus Selector2/1, Bus Selector4/1, Bus Selector6/1
  Bus Creator/1 -> Mz [Nm]/1  "Mz [Nm]"
  Bus Selector6/1 -> Pure Mz RR/4(alpha)  "<Slip Angle RR [deg]>"
  Bus Selector4/1 -> Pure Mz RL/4(alpha)  "<Slip Angle RL [deg]>"
  Tire Forces [N]/1 -> Bus Selector1/1, Bus Selector3/1, Bus Selector5/1, Bus Selector7/1

== system Main/Wheels & Tires/Slip Ratio & Slip Angle Calculation/Slip Angle ==
  X Velocity [m/s] : Inport
  Yaw Rate [rad/s] : Inport  Port=2
  Y Velocity [m/s] : Inport  Port=3
  Steering : Inport  Port=4
  Bus Creator : BusCreator  Inputs=4
  Bus Selector : BusSelector  OutputSignals=Steering Angle FL [rad]
  Bus Selector3 : BusSelector  OutputSignals=Steering Angle FR [rad]
  Bus Selector4 : BusSelector  OutputSignals=Steering Angle RL [rad]
  Bus Selector5 : BusSelector  OutputSignals=Steering Angle RR [rad]
  Slip Angle FL : Subsystem
  Slip Angle FR : Subsystem
  Slip Angle RL : Subsystem
  Slip Angle RR : Subsystem
  Slip Angle [rad] : Outport
  wires:
  Bus Selector5/1 -> Slip Angle RR/4(Steering Angle RR [rad])  "<Steering Angle RR [rad]>"
  Bus Selector4/1 -> Slip Angle RL/4(Steering Angle RL [rad])  "<Steering Angle RL [rad]>"
  Bus Selector3/1 -> Slip Angle FR/4(Steering Angle FR [rad])  "<Steering Angle FR [rad]>"
  Yaw Rate [rad/s]/1 -> Slip Angle FR/3(Yaw Rate [rad/s]), Slip Angle RL/3(Yaw Rate [rad/s]), Slip Angle RR/3(Yaw Rate [rad/s]), Slip Angle FL/3(Yaw Rate [rad/s])
  Y Velocity [m/s]/1 -> Slip Angle RL/2(Y Velocity [m/s]), Slip Angle RR/2(Y Velocity [m/s]), Slip Angle FR/2(Y Velocity [m/s]), Slip Angle FL/2(Y Velocity [m/s])
  X Velocity [m/s]/1 -> Slip Angle FR/1(X Velocity [m/s]), Slip Angle RL/1(X Velocity [m/s]), Slip Angle RR/1(X Velocity [m/s]), Slip Angle FL/1(X Velocity [m/s])
  Slip Angle RR/1(Slip Angle RR [rad]) -> Bus Creator/4  "Slip Angle RR [rad]"
  Slip Angle RL/1(Slip Angle RL [rad]) -> Bus Creator/3  "Slip Angle RL [rad]"
  Slip Angle FR/1(Slip Angle FR [rad]) -> Bus Creator/2  "Slip Angle FR [rad]"
  Slip Angle FL/1(Slip Angle FL [rad]) -> Bus Creator/1  "Slip Angle FL [rad]"
  Bus Creator/1 -> Slip Angle [rad]/1
  Bus Selector/1 -> Slip Angle FL/4(Steering Angle FL [rad])  "<Steering Angle FL [rad]>"
  Steering/1 -> Bus Selector/1, Bus Selector3/1, Bus Selector4/1, Bus Selector5/1

== system Main/Wheels & Tires/Slip Ratio & Slip Angle Calculation/Slip Ratio  ==
  Wheel Speeds [rad/s] : Inport
  X Velocity [m/s] : Inport  Port=2
  Yaw Rate [rad/s] : Inport  Port=3
  Bus Creator : BusCreator  Inputs=4
  Bus Selector : BusSelector  OutputSignals=Wheel Speeds [rad/s].Wheel Speed FL [rad/s],Wheel Speeds [rad/s].Wheel Speed FR [rad/s],Wheel Speeds [rad/s].Wheel Speed RL [rad/s],Wheel Speeds [rad/s].Wheel Speed RR [rad/s]
  Slip ratio FL : Subsystem
  Slip ratio FR : Subsystem
  Slip ratio RL : Subsystem
  Slip ratio RR : Subsystem
  Slip Ratio : Outport
  wires:
  Yaw Rate [rad/s]/1 -> Slip ratio FL/3(Yaw Rate [rad/s]), Slip ratio FR/3(Yaw Rate [rad/s]), Slip ratio RR/3(Yaw Rate [rad/s]), Slip ratio RL/3(Yaw Rate [rad/s])
  X Velocity [m/s]/1 -> Slip ratio FL/2(X Velocity [m/s]), Slip ratio FR/2(X Velocity [m/s]), Slip ratio RL/2(X Velocity [m/s]), Slip ratio RR/2(X Velocity [m/s])
  Slip ratio RR/1(Slip Ratio RR) -> Bus Creator/4  "Slip Ratio RR"
  Slip ratio RL/1(Slip Ratio RL) -> Bus Creator/3  "Slip Ratio RL"
  Slip ratio FR/1(Slip Ratio FR) -> Bus Creator/2  "Slip Ratio FR"
  Slip ratio FL/1(Slip Ratio FL) -> Bus Creator/1  "Slip Ratio FL"
  Bus Selector/4 -> Slip ratio RR/1(Wheel Speed RR [rad/s])  "<Wheel Speed RR [rad/s]>"
  Bus Selector/3 -> Slip ratio RL/1(Wheel Speed RL [rad/s])  "<Wheel Speed RL [rad/s]>"
  Bus Selector/2 -> Slip ratio FR/1(Wheel Speed FR [rad/s])  "<Wheel Speed FR [rad/s]>"
  Bus Selector/1 -> Slip ratio FL/1(Wheel Speed FL [rad/s])  "<Wheel Speed FL [rad/s]>"
  Bus Creator/1 -> Slip Ratio/1
  Wheel Speeds [rad/s]/1 -> Bus Selector/1

== system Main/Wheels & Tires/Wheel Speeds /Rolling Resistance Calculation ==
  Fz [N] : Inport
  Bus Selector : BusSelector  OutputSignals=Fz FL [N],Fz FR [N],Fz RL [N],Fz RR [N]
  Bus Creator : BusCreator  Inputs=4
  Gain{,1,4,6} (4 alike) : Gain  Gain=Tire_radius
  Gain{2..3,5,7} (4 alike) : Gain  Gain=Wheel_rolling_resistance
  Rolling Resistance : Outport
  wires:
  Bus Selector/4 -> Gain6/1  "<Fz RR [N]>"
  Bus Selector/3 -> Gain4/1  "<Fz RL [N]>"
  Bus Selector/2 -> Gain1/1  "<Fz FR [N]>"
  Gain6/1 -> Gain7/1
  Gain4/1 -> Gain5/1
  Gain1/1 -> Gain3/1
  Bus Selector/1 -> Gain/1  "<Fz FL [N]>"
  Fz [N]/1 -> Bus Selector/1
  Bus Creator/1 -> Rolling Resistance/1  "Rolling Resistance"
  Gain7/1 -> Bus Creator/4  "Rolling Resistance RR"
  Gain5/1 -> Bus Creator/3  "Rolling Resistance RL"
  Gain3/1 -> Bus Creator/2  "Rolling Resistance FR"
  Gain2/1 -> Bus Creator/1  "Rolling Resistance FL"
  Gain/1 -> Gain2/1

== system Main/Wheels & Tires/Wheel Speeds /Wheel Speed FL ==
  Rolling Resistance : Inport
  Fx [N] : Inport  Port=2
  Torque [Nm] : Inport  Port=3
  Add1 : Sum  Inputs=--+-
  Bus Selector : BusSelector  OutputSignals=Brake Torque [Nm].Brake Torque FL [Nm],Motor Torque [Nm].Motor Torque FL [Nm]
  Bus Selector1 : BusSelector  OutputSignals=Rolling Resistance FL
  Bus Selector2 : BusSelector  OutputSignals=Fx FL [N]
  Constant4 : Constant  Value=Tire_radius
  Gain : Gain  Gain=Gear_ratio
  Gain1 : Gain  Gain=1/Iz_wheel
  Integrator2 : Integrator  InitialCondition=start_velocity_x / Tire_radius + 3
  Product : Product
  Saturation : Saturate  UpperLimit=200  LowerLimit=-20
  Wheel Speed FL [rad/s] : Outport
  wires:
  Gain/1 -> Add1/3
  Saturation/1 -> Wheel Speed FL [rad/s]/1
  Rolling Resistance/1 -> Bus Selector1/1
  Torque [Nm]/1 -> Bus Selector/1
  Product/1 -> Add1/1
  Constant4/1 -> Product/1
  Bus Selector1/1 -> Add1/4  "<Rolling Resistance FL>"
  Bus Selector/1 -> Add1/2  "<Brake Torque FL [Nm]>"
  Fx [N]/1 -> Bus Selector2/1
  Bus Selector2/1 -> Product/2  "<Fx FL [N]>"
  Gain1/1 -> Integrator2/1
  Integrator2/1 -> Saturation/1
  Add1/1 -> Gain1/1  "Wheel Torque FL [Nm]"
  Bus Selector/2 -> Gain/1  "<Motor Torque FL [Nm]>"

== system Main/Wheels & Tires/Wheel Speeds /Wheel Speed FR ==
  Rolling Resistance : Inport
  Fx [N] : Inport  Port=2
  Torque [Nm] : Inport  Port=3
  Add1 : Sum  Inputs=--+-
  Bus Selector : BusSelector  OutputSignals=Brake Torque [Nm].Brake Torque FR [Nm],Motor Torque [Nm].Motor Torque FR [Nm]
  Bus Selector1 : BusSelector  OutputSignals=Rolling Resistance RL
  Bus Selector2 : BusSelector  OutputSignals=Fx FR [N]
  Constant4 : Constant  Value=Tire_radius
  Gain : Gain  Gain=Gear_ratio
  Gain1 : Gain  Gain=1/Iz_wheel
  Integrator2 : Integrator  InitialCondition=start_velocity_x / Tire_radius + 3
  Product : Product
  Saturation : Saturate  UpperLimit=200  LowerLimit=-20
  Wheel Speed FR [rad/s] : Outport
  wires:
  Gain/1 -> Add1/3
  Saturation/1 -> Wheel Speed FR [rad/s]/1
  Rolling Resistance/1 -> Bus Selector1/1
  Torque [Nm]/1 -> Bus Selector/1
  Product/1 -> Add1/1
  Constant4/1 -> Product/1
  Bus Selector1/1 -> Add1/4  "<Rolling Resistance RL>"
  Bus Selector/1 -> Add1/2  "<Brake Torque FR [Nm]>"
  Fx [N]/1 -> Bus Selector2/1
  Bus Selector2/1 -> Product/2  "<Fx FR [N]>"
  Gain1/1 -> Integrator2/1
  Integrator2/1 -> Saturation/1
  Add1/1 -> Gain1/1
  Bus Selector/2 -> Gain/1  "<Motor Torque FR [Nm]>"

== system Main/Wheels & Tires/Wheel Speeds /Wheel Speed RL ==
  Rolling Resistance : Inport
  Fx [N] : Inport  Port=2
  Torque [Nm] : Inport  Port=3
  Add1 : Sum  Inputs=--+-
  Bus Selector : BusSelector  OutputSignals=Brake Torque [Nm].Brake Torque RL [Nm],Motor Torque [Nm].Motor Torque RL [Nm]
  Bus Selector1 : BusSelector  OutputSignals=Rolling Resistance RL
  Bus Selector2 : BusSelector  OutputSignals=Fx RL [N]
  Constant4 : Constant  Value=Tire_radius
  Gain : Gain  Gain=Gear_ratio
  Gain1 : Gain  Gain=1/Iz_wheel
  Integrator2 : Integrator  InitialCondition=start_velocity_x / Tire_radius + 3
  Product : Product
  Saturation : Saturate  UpperLimit=200  LowerLimit=-20
  Wheel Speed RL [rad/s] : Outport
  wires:
  Gain/1 -> Add1/3
  Bus Selector/2 -> Gain/1  "<Motor Torque RL [Nm]>"
  Constant4/1 -> Product/1
  Add1/1 -> Gain1/1
  Product/1 -> Add1/1
  Integrator2/1 -> Saturation/1
  Gain1/1 -> Integrator2/1
  Bus Selector/1 -> Add1/2  "<Brake Torque RL [Nm]>"
  Bus Selector1/1 -> Add1/4  "<Rolling Resistance RL>"
  Torque [Nm]/1 -> Bus Selector/1
  Saturation/1 -> Wheel Speed RL [rad/s]/1
  Rolling Resistance/1 -> Bus Selector1/1
  Bus Selector2/1 -> Product/2  "<Fx RL [N]>"
  Fx [N]/1 -> Bus Selector2/1

== system Main/Wheels & Tires/Wheel Speeds /Wheel Speed RR ==
  Rolling Resistance : Inport
  Fx [N] : Inport  Port=2
  Torque [Nm] : Inport  Port=3
  Add1 : Sum  Inputs=--+-
  Bus Selector : BusSelector  OutputSignals=Brake Torque [Nm].Brake Torque RR [Nm],Motor Torque [Nm].Motor Torque RR [Nm]
  Bus Selector1 : BusSelector  OutputSignals=Rolling Resistance RR
  Bus Selector2 : BusSelector  OutputSignals=Fx RR [N]
  Constant4 : Constant  Value=Tire_radius
  Gain : Gain  Gain=Gear_ratio
  Gain1 : Gain  Gain=1/Iz_wheel
  Integrator2 : Integrator  InitialCondition=start_velocity_x / Tire_radius + 3
  Product : Product
  Saturation : Saturate  UpperLimit=200  LowerLimit=-20
  Wheel Speed RL [rad/s] : Outport
  wires:
  Gain/1 -> Add1/3
  Saturation/1 -> Wheel Speed RL [rad/s]/1
  Rolling Resistance/1 -> Bus Selector1/1
  Torque [Nm]/1 -> Bus Selector/1
  Product/1 -> Add1/1
  Constant4/1 -> Product/1
  Bus Selector1/1 -> Add1/4  "<Rolling Resistance RR>"
  Bus Selector/1 -> Add1/2  "<Brake Torque RR [Nm]>"
  Fx [N]/1 -> Bus Selector2/1
  Bus Selector2/1 -> Product/2  "<Fx RR [N]>"
  Gain1/1 -> Integrator2/1
  Integrator2/1 -> Saturation/1
  Add1/1 -> Gain1/1
  Bus Selector/2 -> Gain/1  "<Motor Torque RR [Nm]>"

== system Main/Powertrain/Motors/Control Algorithms/TV Algorithm ==
  Torque Command [Nm] : Inport
  Wheel Speed [rad/s] : Inport  Port=2
  Terminator : Terminator
  Commanded Torque FL [Nm] : Outport
  Commanded Torque FR [Nm] : Outport  Port=2
  Commanded Torque RL [Nm] : Outport  Port=3
  Commanded Torque RR [Nm] : Outport  Port=4
  wires:
  Wheel Speed [rad/s]/1 -> Terminator/1
  Torque Command [Nm]/1 -> Commanded Torque RL [Nm]/1, Commanded Torque RR [Nm]/1, Commanded Torque FL [Nm]/1, Commanded Torque FR [Nm]/1
